simulink model "satelliteProject"  (R2013a)
settings: Solver=ode45  StartTime=0.0  StopTime=10.0  MaxStep=1e-3  RelTol=1e-5
values from neighbouring files (symbols this model uses):
  ditherAmp = handles.ditherAmplitude    [E205AdaptiveControl_GK_LPJ.m]
  J = 2    [finalproject.m]
  Jhat = 1    [finalproject.m]
  mud = 10    [finalproject.m]
  mup = 10    [finalproject.m]
  omega = 10    [E205AdaptiveControl_GK_LPJ.m]    (also in finalproject.m)
  zeta = 1    [E205AdaptiveControl_GK_LPJ.m]    (also in finalproject.m)
undefined symbols (not defined in the file or in its folder): Amplitude, ditherFreq, Frequency, initialAngle, initialVelocity, inputChoice, Period
libraries: simulink x1
settings Model: Creator=molinder  LastModifiedBy=gkhadge
settings DataIOCC: SignalLoggingSaveFormat=ModelDataLogs
settings OptimizationCC: ExpressionDepthLimit=2147483647
settings DebuggingCC: FcnCallInpInsideContextMsg=EnableAllAsWarning

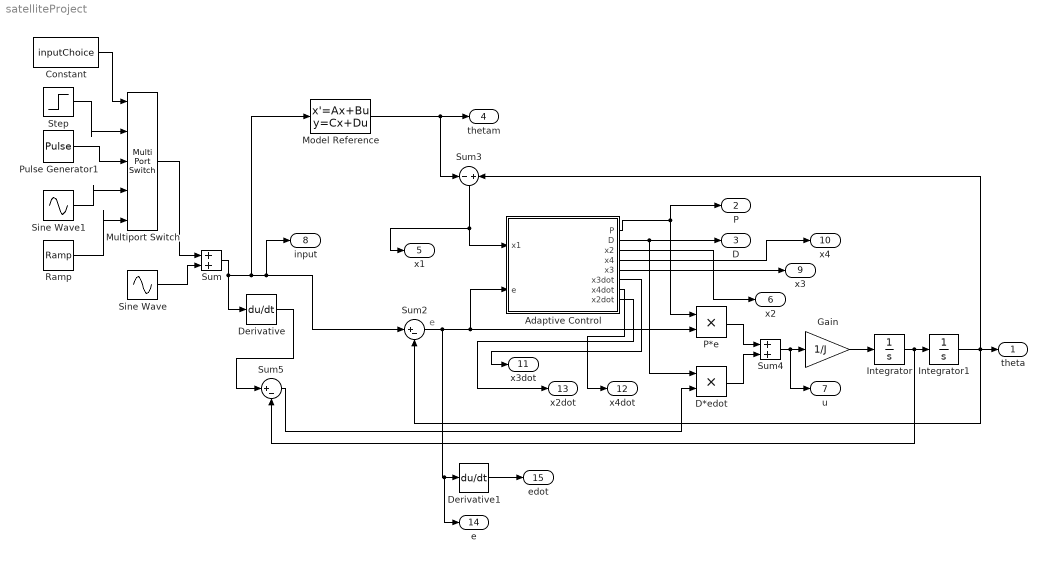
== system satelliteProject ==
  note: e
  Adaptive Control : Subsystem
  Constant : Constant  Value=inputChoice
  D*edot : Product
  Derivative : Derivative
  Derivative1 : Derivative
  Gain : Gain  Gain=1/J
  Integrator : Integrator  InitialCondition=initialVelocity
  Integrator1 : Integrator  InitialCondition=initialAngle
  Model Reference : StateSpace  A=[-20 -100; 1 0]  B=[100;0]  C=[0 1]  D=0  X0=[initialVelocity initialAngle]
  Multiport Switch : MultiPortSwitch  Inputs=4
  P*e : Product
  Pulse Generator1 : DiscretePulseGenerator  PulseType=Time based  Amplitude=Amplitude  Period=Period  PulseWidth=50
  Ramp : simulink/Sources/Ramp  slope=Amplitude  start=0  X0=0
  Sine Wave : Sin  Amplitude=ditherAmp  Frequency=ditherFreq  SampleTime=0
  Sine Wave1 : Sin  Amplitude=Amplitude  Frequency=Frequency  SampleTime=0
  Step : Step  After=Amplitude  SampleTime=0
  Sum : Sum
  Sum2 : Sum  Inputs=|+-
  Sum3 : Sum  Inputs=-+
  Sum4 : Sum
  Sum5 : Sum  Inputs=|+-
  theta : Outport
  P : Outport  Port=2
  D : Outport  Port=3
  thetam : Outport  Port=4
  x1 : Outport  Port=5
  x2 : Outport  Port=6
  u : Outport  Port=7
  input : Outport  Port=8
  x3 : Outport  Port=9
  x4 : Outport  Port=10
  x3dot : Outport  Port=11
  x4dot : Outport  Port=12
  x2dot : Outport  Port=13
  e : Outport  Port=14
  edot : Outport  Port=15
  wires:
  Model Reference/1 -> Sum3/1, thetam/1
  Sum3/1 -> x1/1, Adaptive Control/1(x1)
  Sum2/1 -> e/1, Derivative1/1, Adaptive Control/2(e), P*e/2
  Sum4/1 -> u/1, Gain/1
  D*edot/1 -> Sum4/2
  P*e/1 -> Sum4/1
  Sum5/1 -> D*edot/2
  Gain/1 -> Integrator/1
  Integrator/1 -> Sum5/2, Integrator1/1
  Integrator1/1 -> Sum3/2, Sum2/2, theta/1
  Adaptive Control/1(P) -> P*e/1, P/1
  Adaptive Control/2(D) -> D*edot/1, D/1
  Adaptive Control/3(x2) -> x2/1
  Sum/1 -> Model Reference/1, input/1, Sum2/1, Derivative/1
  Derivative/1 -> Sum5/1
  Sine Wave/1 -> Sum/2
  Constant/1 -> Multiport Switch/1
  Multiport Switch/1 -> Sum/1
  Step/1 -> Multiport Switch/2
  Pulse Generator1/1 -> Multiport Switch/3
  Sine Wave1/1 -> Multiport Switch/4
  Ramp/1 -> Multiport Switch/5
  Adaptive Control/5(x3) -> x3/1
  Adaptive Control/4(x4) -> x4/1
  Adaptive Control/6(x3dot) -> x3dot/1
  Adaptive Control/7(x4dot) -> x4dot/1
  Adaptive Control/8(x2dot) -> x2dot/1
  Derivative1/1 -> edot/1

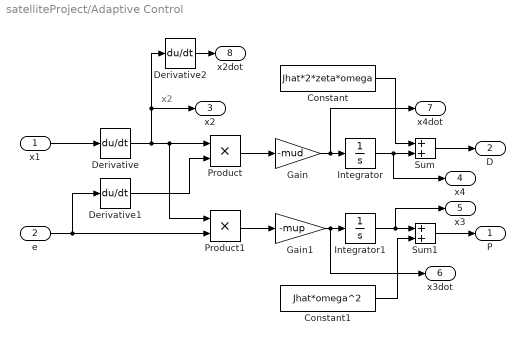
== system satelliteProject/Adaptive Control ==
  note: x2
  x1 : Inport
  e : Inport  Port=2
  Constant : Constant  Value=Jhat*2*zeta*omega
  Constant1 : Constant  Value=Jhat*omega^2
  Derivative : Derivative
  Derivative1 : Derivative
  Derivative2 : Derivative
  Gain : Gain  Gain=-mud
  Gain1 : Gain  Gain=-mup
  Integrator : Integrator
  Integrator1 : Integrator
  Product : Product
  Product1 : Product
  Sum : Sum
  Sum1 : Sum
  P : Outport
  D : Outport  Port=2
  x2 : Outport  Port=3
  x4 : Outport  Port=4
  x3 : Outport  Port=5
  x3dot : Outport  Port=6
  x4dot : Outport  Port=7
  x2dot : Outport  Port=8
  wires:
  x1/1 -> Derivative/1
  e/1 -> Product1/2, Derivative1/1
  Derivative/1 -> Derivative2/1, x2/1, Product1/1, Product/1
  Derivative1/1 -> Product/2
  Product1/1 -> Gain1/1
  Product/1 -> Gain/1
  Gain/1 -> x4dot/1, Integrator/1
  Gain1/1 -> x3dot/1, Integrator1/1
  Constant/1 -> Sum/1
  Integrator/1 -> x4/1, Sum/2
  Sum/1 -> D/1
  Integrator1/1 -> x3/1, Sum1/1
  Sum1/1 -> P/1
  Constant1/1 -> Sum1/2
  Derivative2/1 -> x2dot/1
